simulink model "LAB6T4"  (R2018b)
settings: Solver=ode113  StartTime=0.0  StopTime=100  MaxStep=0.07  RelTol=1e-1
libraries: aerolibanim x1
settings Model: Creator=aloisia  LastModifiedBy=aloisia

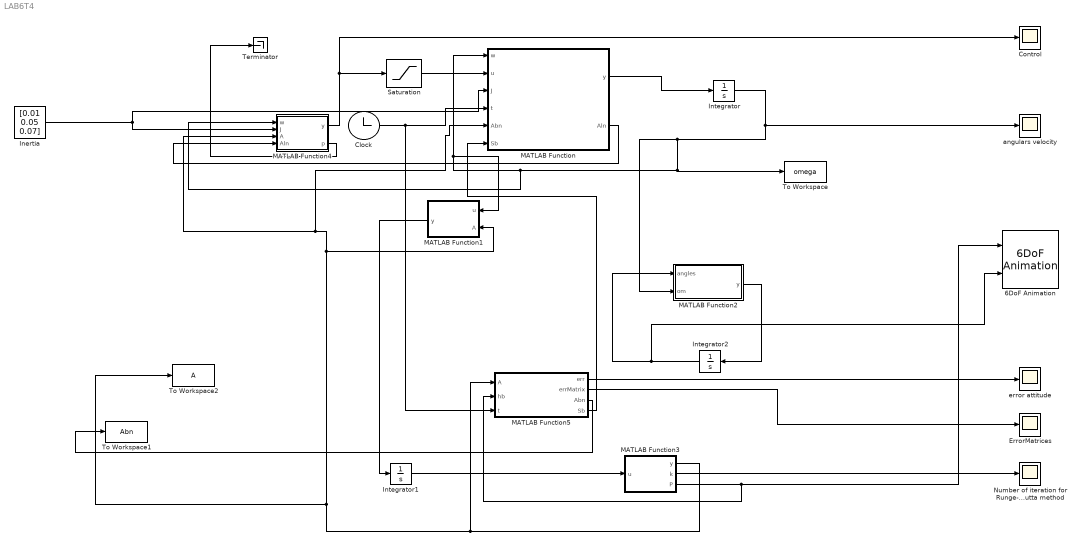
== system LAB6T4 ==
  6DoF Animation : aerolibanim/6DoF Animation  u1=[0 4000 -2000 2000 -5000 -3000]  u2=0.07  u3=800  u4=[4000 0 -5000]  u5=Fixed position  u6=[2000 500 -3150]  u7=10  u8=on
      settings: SourceProductName=Aerospace Blockset
  Clock : Clock
  Control : Scope
  "ErrorMatrices " : Scope
  "Inertia " : Constant  Tag=J  Description=J  Value=[0.01 0.05 0.07]
  Integrator : Integrator  InitialCondition=[0.01;0.01;0.03]
  Integrator1 : Integrator  InitialCondition=[-0.782 0 -0.6233; 0.6233 0 -0.782; 0 -1 0]
  Integrator2 : Integrator  InitialCondition=[0;0;0]
  MATLAB Function : MATLAB Function  TreatAsAtomicUnit=on
  MATLAB Function1 : MATLAB Function  TreatAsAtomicUnit=on
  MATLAB Function2 : MATLAB Function  TreatAsAtomicUnit=on
  MATLAB Function3 : MATLAB Function  TreatAsAtomicUnit=on
  MATLAB Function4 : MATLAB Function  TreatAsAtomicUnit=on
  MATLAB Function5 : MATLAB Function  TreatAsAtomicUnit=on
  Number of iteration for Runge-Kutta method : Scope
  Saturation : Saturate  UpperLimit=0.1  LowerLimit=-0.1  LinearizeAsGain=off  ZeroCross=off
  Terminator : Terminator
  To Workspace : ToWorkspace  VariableName=omega  SampleTime=-1
  To Workspace1 : ToWorkspace  VariableName=Abn  SampleTime=-1
  To Workspace2 : ToWorkspace  VariableName=A  SampleTime=-1
  "angulars velocity " : Scope
  error attitude : Scope
  wires:
  Integrator/1 -> MATLAB Function2/2(om), To Workspace/1, MATLAB Function4/1(w), MATLAB Function/1(w), MATLAB Function1/1(u), "angulars velocity "/1
  "Inertia "/1 -> MATLAB Function/3(J), MATLAB Function4/2(J)
  MATLAB Function/1(y) -> Integrator/1
  Clock/1 -> MATLAB Function5/3(t), MATLAB Function/4(t)
  Integrator1/1 -> MATLAB Function3/1(u)
  MATLAB Function3/2(k) -> Number of iteration for Runge-Kutta method/1
  MATLAB Function4/1(y) -> Saturation/1, Control/1
  MATLAB Function1/1(y) -> Integrator1/1
  MATLAB Function3/1(y) -> MATLAB Function5/1(A), To Workspace2/1, MATLAB Function/5(Abn), MATLAB Function4/3(A), MATLAB Function1/2(A)
  MATLAB Function3/3(P) -> MATLAB Function5/2(hb), 6DoF Animation/1
  MATLAB Function2/1(y) -> Integrator2/1
  Integrator2/1 -> 6DoF Animation/2, MATLAB Function2/1(angles)
  MATLAB Function/2(Aln) -> MATLAB Function4/4(Aln)
  Saturation/1 -> MATLAB Function/2(u)
  MATLAB Function5/1(err) -> error attitude/1
  MATLAB Function5/3(Abn) -> To Workspace1/1
  MATLAB Function5/4(Sb) -> MATLAB Function/6(Sb)
  MATLAB Function5/2(errMatrix) -> "ErrorMatrices "/1
  MATLAB Function4/2(p) -> Terminator/1

== matlab function LAB6T4/MATLAB Function1 ==
  data: u input; y output; A input
function y = kinematics(u,A)


W=[0 -u(3) u(2); u(3) 0 -u(1); -u(2) -u(1) 0];

Adot=-W*A ;

y=Adot ;
end

== matlab function LAB6T4/MATLAB Function ==
  data: w input; u input; y output; J input; t input; Abn input; Aln output; Sb input
function [y,Aln] = euler(w,u,J,t,Abn,Sb)

%Set Data

Ix=J(1); Iy=J(2); Iz=J(3) ;
wx=w(1) ; wy=w(2); wz=w(3);
wdot=zeros(3,1);

%%Gravity Gradient

R=42168;                    %Geostationary orbit
n=(398600/(R^3))^0.5 ;      %Angular velocity for circular orbit
Aln=[cos(n*t) sin(n*t) 0 ; -sin(n*t) cos(n*t) 0; 0 0 1];
Abl=Abn*(Aln');
c=Abl*[1;0;0];
Ma1=(3*(n^2))*((Iz-Iy)*c(3)*c(2)) ;
Ma2=(3*(n^2))*((Ix-Iz)*c(1)*c(3)) ;
Ma3=(3*(n^2))*((Iy-Ix)*c(1)*c(2));
% SRP disturbance
n1=[1;0;0]; n4=-n1;
n2=[0;1;0]; n5=-n2;
n3=[0;0;1]; n6=-n3;

N =[n1 n2 n3 n4 n5 n6];

a=0.50;                 %[m]                                    
A = a*2;                %[m^2]
P = 1358/(300000*1e3);  %[W/m^2]/[m/s]
rho_s=0.5;              %[kg/m^3]
rho_d=0.1;              %[kg/m^3]
F = zeros(3,6);
br=(a/2).*N;
M=zeros(3,6);


for i = 1:6
    
    if dot(Sb,N(:,i))>0
        F(:,i)= P*A * dot(Sb,N(:,i)) * ((1-rho_s)*Sb + (2*rho_s *dot(Sb,N(:,i))...
            + 2/3 * rho_d)* N(:,i));
    else
        F(:,i) = zeros(3,1);
     
    end
  M(:,i)=cross(F(:,i),br(:,i));  
end

M=M';
Mt=sum(M(:,1:3));



%% Euler Equation
wdot(1)= ((Iy-Iz)/Ix)*wy*wz+u(1)/Ix+Ma1/Ix+Mt(1)/Ix;
wdot(2)= ((Iz-Ix)/Iy)*wx*wz+u(2)/Iy+Ma2/Iy+Mt(2)/Iy;
wdot(3)= ((Ix-Iy)/Iz)*wx*wy+u(3)/Iz+Ma3/Iz+Mt(3)/Iz;


y = wdot;
Aln = Aln;
end

== matlab function LAB6T4/MATLAB Function2 ==
  data: angles input; y output; om input
function y = fcn(angles,om)

% This function provides the calculation of A by using 
% Phi, theta, psi and omega.Radiants
phi = angles(1);
theta = angles(2);
psi = angles(3);

phidot = (om(1)*cos(psi) - om(2)*sin(psi)) / cos(theta);
thetadot = om(2)*cos(psi) + om(1)*sin(psi);
psidot = om(3) - (om(1)*cos(psi) - om(2)*sin(psi))* sin(theta)/cos(theta);
anglesdot = [phidot; thetadot; psidot];

y = anglesdot;
end

== matlab function LAB6T4/MATLAB Function3 ==
  data: u input; y output; k output; P output
function [y,k,P]  = ortho(u)

c=1; A=u; k=0;
while c>0.000001

A=(1.5.*A)-(A*(A')*A./2) ; % Runge-Kutta method
c=trace((eye(3)-(A')*A)) ; % error
k=k+1 ; %counter
end

z=k;
y=A ;
P = A * [1;0;0];

end

== matlab function LAB6T4/MATLAB Function4 ==
  data: w input; y output; J input; A input; Aln input; p output
function [y,p] = control(w,J,A,Aln)

% set gain
k1=0.5; k2=0.5;

% control law 
Jd=diag(J); 
K1=k1*Jd ; K2=k2*Jd;
Ad=Aln;
%Ad = eye(3);
Ae=A*Ad' ;
Q=(Ae')-Ae ;
e=[Q(3,2) Q(1,3) Q(2,1)]';
% Circular orbits are considered

 R=42168;
 n=(398600/(R^3))^0.5 ;
 wln = [0;0;n];
 we = w - Ae*wln;
 
u=-K1*we-K2*e;

y=u;
p=A'*[0; 0; 1];
end

== matlab function LAB6T4/MATLAB Function5 ==
  data: A input; err output; errMatrix output; hb input; t input; Abn output; Sb output
function [err,errMatrix,Abn,Sb] = attitude_pointing(A,hb,t)
    %LAB 6: TASK 3
    %Circular orbit is considered
    
    n=2*pi/(365.25*3600*24);    % Mean motion
    B=pi/6+150*n;               % Initial phase (150s from previous detumbling)
    ep=23.45*pi/180;            % Ecliptic inclination
    
    % Sun pointing vector
    Sn=[cos(n*t+B); sin(n*t+B)*cos(ep); sin(n*t+B)*sin(ep)];
    
    % Earth horizon pointing vector
    hn = -[cos(n*t) sin(n*t) 0]';
    % hb=A*hn; %reconstruction by attitude
    %Accuracy error
    es = 1/60 * pi/180;
    ee = 6/60 * pi/180;
    Aes = [cos(es)*cos(es) cos(es)*sin(es)*sin(es)+sin(es)*cos(es) -cos(es)*sin(es)*cos(es)+sin(es)*sin(es);...
          -sin(es)*cos(es) -sin(es)*sin(es)*sin(es)+cos(es)*cos(es) sin(es)*sin(es)*cos(es)+cos(es)*sin(es);...
          sin(es) -cos(es)*sin(es) cos(es)*cos(es)];
      
    Aee = [cos(ee)*cos(ee) cos(ee)*sin(ee)*sin(ee)+sin(ee)*cos(ee) -cos(ee)*sin(ee)*cos(ee)+sin(ee)*sin(ee);...
      -sin(ee)*cos(ee) -sin(ee)*sin(ee)*sin(ee)+cos(ee)*cos(ee) sin(ee)*sin(ee)*cos(ee)+cos(ee)*sin(ee);...
      sin(ee) -cos(ee)*sin(ee) cos(ee)*cos(ee)];
  
    %Sensors data
    hb =  hb/norm(hb);
    hb_noerr = hb/norm(hb);
    Sb =  A*Sn/norm(A*Sn);
    Sb_noerr =  A*Sn/norm(A*Sn);
    

    SbXhb = cross(Sb,hb);
    SnXhn = cross(Sn,hn);
    Vb = [ Sb  SbXhb/norm(SbXhb) cross(Sb,SbXhb/norm(SbXhb))]; 
    Vn = [ Sn  SnXhn/norm(SnXhn) cross(Sn,SnXhn/norm(SnXhn))]; 
    Abn = Vb*Vn';
    
   errMatrix= abs(A - Abn);
   err = abs(norm(Sb - Abn*Sn));
   
end
